simulink model "RefModel_Task"  (R2015b)
settings: configuration reference "CenterOutReachConfigSet" (kept outside this file)
undefined symbols (not defined in the file or in its folder): SimulinkParameter_TunableConditionRepeats, SimulinkParameter_TunableConditions, SimulinkParameter_TunableDataLoggerInfo, SimulinkParameter_TunableNextTrialId, SimulinkParameter_TunableParam, SimulinkParameter_TunableTaskControl
libraries: libBusSerialize x7, libUtilities x1, dspsrcs4 x1
(part 2 of 3)

== stateflow chart RefModel_Task/Task Stateflow ==
  state TaskTimeoutContainer [parallel]
    settings: executionOrder=1
    state TaskNotRunning
      en:
      TD.taskRunning = uint8(0);
      JuiceRelease = uint8(0);
      if TaskControl.controlImaging
      % if we were imaging, pause it
      scopeCommand = ScopeCommand.StopImaging;
      send(SendScope);
      end
      ex:
      TD.taskRunning = uint8(1);
      state TaskPaused
        en:
        state = TaskState.TaskPaused;
        displayCommand = DisplayCommand.TaskPaused;
        send(SendDisplay);
      state TaskPurgatory
        en:
        TD.inPurgatory = uint8(1);
        TD.purgatoryTimeRemaining = P.purgatoryTime;
        state = TaskState.TaskPurgatory;
        TD.consecutiveNoStarts = uint16(0);
        displayCommand = DisplayCommand.TaskTimeout;
        send(SendDisplay);
        du:
        TD.purgatoryTimeRemaining = TD.purgatoryTimeRemaining - uint32(1);
        ex:
        TD.inPurgatory = uint8(0);
    state Task
      state TaskFlow [parallel]
        du:
        computeHandState();
        ex:
        send(AbortJuice, JuiceToggle);
        settings: executionOrder=1
        state InitTrial
          en:
          send(TrialStart);
          send(PhotoboxReset, PhotoboxEvents);
          TD.taskRunning = uint8(1);
          % this counter will be reset to zero when the appropriate
          % point in the trial has been reached
          TD.consecutiveNoStarts = TD.consecutiveNoStarts + uint16(1);
          displayCommand = DisplayCommand.InitTrial;
          send(SendDisplay);
          if C.hasImaging && TaskControl.controlImaging
          TD.imagingThisTrial = uint8(1);
          scopeCommand = ScopeCommand.NextTrial;
          send(SendScope);
          scopeCommand = ScopeCommand.StartImagingOnTrigger;
          send(SendScope);
          else
          TD.imagingThisTrial = uint8(0);
          end
          state = TaskState.InitTrial;
          resetTrialData();
        state StartTask
          en:
          state = TaskState.StartTask;
          displayCommand = DisplayCommand.StartTask;
          send(SendDisplay);
        state CenterAcquireHold
          state CenterAcquireLogic [parallel]
            settings: executionOrder=1
            state WaitCenterAcquire
              en:
              state = TaskState.WaitCenterAcquire;
              displayCommand = DisplayCommand.CenterOnset;
              send(SendDisplay);
              eventCode = TaskEvent.CenterOnset;
              send(SendEvent);
            state WaitCenterSettle
              en:
              state = TaskState.WaitCenterSettle;
              displayCommand = DisplayCommand.CenterAcquired;
              send(SendDisplay);
              eventCode = TaskEvent.CenterAcquired;
              send(SendEvent);
              ex:
              % Establish hold window for td.isHolding
              TD.holdXCenter = HandBus.handX;
              TD.holdYCenter = HandBus.handY;
            state CenterUnacquire
              en: displayCommand = DisplayCommand.CenterUnacquired;
              send(SendDisplay);
              eventCode = TaskEvent.CenterUnacquired;
              send(SendEvent);
            state WaitCenterHold
              en:
              state = TaskState.WaitCenterHold;
              displayCommand = DisplayCommand.CenterSettled;
              send(SendDisplay);
              eventCode = TaskEvent.CenterSettled;
              send(SendEvent);
              % trigger imaging just before TargetOnset
              on after(P.timeCenterHold - P.timeImagingStartBeforeTargetOnset, tick):
              if TD.imagingThisTrial
              scopeCommand = ScopeCommand.StartTrialImaging;
              send(SendScope);
              end
            state CenterHeld
              en:
              displayCommand = DisplayCommand.CenterHeld;
              send(SendDisplay);
              eventCode = TaskEvent.CenterHeld;
              send(SendEvent);
              if P.timeJuiceCenter > 0
              TD.juiceNumDrops = uint16(1);
              TD.juiceDropSize = uint16(P.timeJuiceCenter);
              send(SendJuice, JuiceToggle);
              end
            WaitCenterAcquire -> WaitCenterSettle [order 1] : [TD.isTouchingCenter == 1]
            CenterUnacquire -> WaitCenterAcquire
            WaitCenterSettle -> WaitCenterHold : after(P.timeCenterSettle,tick)
                | % Wait for settling before enforcing hold
            (junction 2183) -> CenterUnacquire [order 2]
            (junction 2186) -> CenterUnacquire [order 2]
            WaitCenterHold -> (junction 2183) [order 1] : [~HandBus.handSeen]
                | % Missing hand position
            WaitCenterHold -> (junction 2186) [order 3] : [~TD.isHoldingCenter]
                | % Moved during center hold = hold - 1> fail trial
            WaitCenterHold -> CenterHeld [order 2] : after(P.timeCenterHold,tick)
                | % Held center
        state ForceNewCondition
          en:
          TD.getNewTrialParams = uint8(1);
        state TrialFailure
          en:
          TD.success = uint8(0);
          if TD.imagingThisTrial
          scopeCommand = ScopeCommand.EndTrialImaging;
          send(SendScope);
          end
          state FailureCenterAcquire % never got to center
            en:
            TD.substantiveFailure = uint8(0);
            TD.getNewTrialParams = uint8(0);
            state = TaskState.FailureCenterAcquire;
            displayCommand = DisplayCommand.FailureCenterFlyAway;
            send(SendDisplay);
            eventCode = TaskEvent.FailureToAcquireCenter;
            send(SendEvent);
          state FailureComputeITI
            en:
            if P.repeatUntilSuccess
            TD.getNewTrialParams = uint8(0);
            end
            TD.failureCode = state;
            computeFailureITI();
            % print failure message to screen
            coder.ceval('printf', ['Failure: %s' 10 0], ...
            [enumToString_TaskState(state) uint8(0)]);
          state FailureHandNotSeen % lost hand position during trial
            en:
            TD.substantiveFailure = uint8(0);
            TD.getNewTrialParams = uint8(1);
            state = TaskState.FailureHandNotSeen;
            displayCommand = DisplayCommand.FailureCenterFlyAway;
            send(SendDisplay);
            eventCode = TaskEvent.FailureHandNotSeen;
            send(SendEvent);
            % print warning message to screen
            coder.ceval('printf', ['WARNING: HAND NOT SEEN' 10 0]);
          state FailureCenterHold % moved while holding
            en:
            TD.substantiveFailure = uint8(0);
            TD.getNewTrialParams = uint8(0);
            state = TaskState.FailureCenterHold;
            displayCommand = DisplayCommand.FailureCenterFlyAway;
            send(SendDisplay);
            eventCode = TaskEvent.FailureBrokeCenterHold;
            send(SendEvent);
          state FailureDelayMove % moved during delay
            en:
            TD.substantiveFailure = uint8(0);
            TD.getNewTrialParams = uint8(1);
            state = TaskState.FailureDelayMove;
            displayCommand = DisplayCommand.FailureTargetFlyAway;
            send(SendDisplay);
            eventCode = TaskEvent.FailureBrokeCenterHoldDelay;
            send(SendEvent);
          state FailureRTTooFast % moved too early post go-cue
            en:
            TD.substantiveFailure = uint8(0);
            TD.getNewTrialParams = uint8(1);
            state = TaskState.FailureRTTooFast;
            displayCommand = DisplayCommand.FailureTargetFlyAway;
            send(SendDisplay);
            eventCode = TaskEvent.FailureRTTooFast;
            send(SendEvent);
          state FailureRTTooSlow % didn't move early enough post go-cue
            en:
            TD.substantiveFailure = uint8(0);
            TD.getNewTrialParams = uint8(1);
            state = TaskState.FailureRTTooSlow;
            displayCommand = DisplayCommand.FailureTargetFlyAway;
            send(SendDisplay);
            eventCode = TaskEvent.FailureRTTooSlow;
            send(SendEvent);
          state FailureTargetAcquire % didn't get target in time
            en:
            TD.substantiveFailure = uint8(1);
            TD.getNewTrialParams = uint8(1);
            state = TaskState.FailureTargetAcquire;
            displayCommand = DisplayCommand.FailureTargetFlyAway;
            send(SendDisplay);
            eventCode = TaskEvent.FailureToAcquireTarget;
            send(SendEvent);
          state FailureTargetHold % moved while holding target
            en:
            TD.substantiveFailure = uint8(1);
            TD.getNewTrialParams = uint8(1);
            state = TaskState.FailureTargetHold;
            displayCommand = DisplayCommand.FailureTargetFlyAway;
            send(SendDisplay);
            eventCode = TaskEvent.FailureToAcquireTarget;
            send(SendEvent);
          state FailurePeakVelocityTooLow % reach too slow
            en:
            TD.substantiveFailure = uint8(1);
            TD.getNewTrialParams = uint8(1);
            state = TaskState.FailureLowPeakVelocity;
            displayCommand = DisplayCommand.FailureTargetFlyAway;
            send(SendDisplay);
            eventCode = TaskEvent.FailureLowPeakVelocity;
            send(SendEvent);
          FailureCenterAcquire % never got to center -> (junction 1353)
          (junction 1353) -> FailureComputeITI : after(1,tick)
          FailureHandNotSeen % lost hand position during trial -> (junction 1353)
          FailurePeakVelocityTooLow % reach too slow -> (junction 1353)
          FailureCenterHold % moved while holding -> (junction 1353)
          FailureDelayMove % moved during delay -> (junction 1353)
          FailureTargetHold % moved while holding target -> (junction 1353)
          FailureRTTooFast % moved too early post go-cue -> (junction 1353)
          FailureRTTooSlow % didn't move early enough post go-cue -> (junction 1353)
          FailureTargetAcquire % didn't get target in time -> (junction 1353)
        state DelayPeriodGoCue
          state GoCue
            state GoCueZeroDelay
              en:
              state = TaskState.GoCueZeroDelay;
              TD.timeTargetOnsetCommand = GlobalClock;
              TD.timeGoCueCommand = GlobalClock;
              displayCommand = DisplayCommand.GoCueZeroDelay;
              send(SendDisplay);
              eventCode = TaskEvent.TargetOnsetCommand;
              send(SendEvent);
              eventCode = TaskEvent.GoCueCommand;
              send(SendEvent);
            state GoCueNonZeroDelay
              en:
              state = TaskState.GoCueNonZeroDelay;
              TD.timeGoCueCommand = GlobalClock;
              displayCommand = DisplayCommand.GoCueNonZeroDelay;
              send(SendDisplay);
              eventCode = TaskEvent.GoCueCommand;
              send(SendEvent);
          state SetTargetInfo
            en:
            TD.targetXCurrent = C.targetX;
            TD.targetYCurrent = C.targetY;
            TD.targetSizeCurrent = C.targetSize;
          state DelayPeriod
            en:
            state = TaskState.DelayPeriod;
            TD.timeTargetOnsetCommand = GlobalClock;
            displayCommand = DisplayCommand.DelayPeriodStart;
            send(SendDisplay);
            eventCode = TaskEvent.TargetOnsetCommand;
            send(SendEvent);
          state WaitMoveOnset
            en:
            state = TaskState.WaitMoveOnset;
            if P.imageDecoderDebugDisplayMode
            end
            du:
            TD.rt = GlobalClock - TD.timeGoCue; % detected by photobox
            TD.rtNominal = GlobalClock - TD.timeGoCueCommand; % not detected by photobox
            ex:
            TD.timeMove = GlobalClock;
            TD.rt = GlobalClock - TD.timeGoCue; % not detected by photobox
            TD.rtNominal = GlobalClock - TD.timeGoCueCommand; % not detected by photobox
            displayCommand = DisplayCommand.MoveOnset;
            send(SendDisplay)
            eventCode = TaskEvent.MoveOnsetOnline;
            send(SendEvent);
          (default) -> SetTargetInfo
          SetTargetInfo -> GoCueZeroDelay [order 1] : [~C.hasCenterTouch || C.delayNominal == 0]
              | % Target Only Zero Delay
          SetTargetInfo -> DelayPeriod [order 2] : % Non-zero Delay
          DelayPeriod -> GoCueNonZeroDelay [order 2] : after(C.delayNominal, tick)
              | % Delay period over
          GoCue -> WaitMoveOnset : after(1,tick)
          WaitMoveOnset -> (junction 1269) [order 2] : [~TD.isHoldingCenter]
              | % Move from center
        state RequestNewTrial
          en: send(GetNewTrial);
        state TargetAcquireHold
          state WaitTargetAcquire
            en:
            state = TaskState.WaitTargetAcquire;
          state WaitTargetSettle
            en:
            % count as initiated the trial (for ~hasCenterTouch)
            TD.consecutiveNoStarts = uint16(0);
            state = TaskState.WaitTargetSettle;
            displayCommand = DisplayCommand.TargetAcquired;
            send(SendDisplay);
            eventCode = TaskEvent.TargetAcquired;
            send(SendEvent);
          state TargetUnacquire
            en: displayCommand = DisplayCommand.TargetUnacquired;
            send(SendDisplay);
            eventCode = TaskEvent.TargetUnacquired;
            send(SendEvent);
          state WaitTargetHold
            en:
            % Establish the hold window around current hand pos
            TD.holdXTarget = HandBus.handX;
            TD.holdYTarget = HandBus.handY;
            state = TaskState.WaitTargetHold;
            % Send TargetSettled
            displayCommand = DisplayCommand.TargetSettled;
            send(SendDisplay);
            eventCode = TaskEvent.TargetSettled;
            send(SendEvent);
            % optionally juice during target hold
            if C.juiceDuringTargetHold
            TD.juiceNumDrops = uint16(50);
            TD.juiceDropSize = uint16(P.targetHoldJuiceSize);
            TD.juiceDropInterval = uint16(P.targetHoldJuiceInterval);
            send(SendJuice, JuiceToggle);
            end
            ex:
            displayCommand = DisplayCommand.TargetHeld;
            send(SendDisplay);
            eventCode = TaskEvent.TargetHeld;
            send(SendEvent);
            send(AbortJuice, JuiceToggle);
          WaitTargetAcquire -> WaitTargetSettle [order 2] : [TD.isTouchingTarget]
              | % Target Acquired
          TargetUnacquire -> WaitTargetAcquire
          (junction 2191) -> TargetUnacquire [order 2] : % allow target reacquire
          WaitTargetSettle -> WaitTargetHold : after(P.timeTargetSettle, tick)
          WaitTargetHold -> (junction 2191) [order 2] : [~TD.isHoldingTarget]
              | % Moved during TargetHold
        state ITI
          en:
          send(TrialEnd);
          state = TaskState.ITI;
          displayCommand = DisplayCommand.ITI;
          send(SendDisplay);
          send(TrialITI);
        state Success
          en:
          state = TaskState.Success;
          TD.success = uint8(1);
          TD.getNewTrialParams = uint8(1);
          if TD.imagingThisTrial
          scopeCommand = ScopeCommand.EndTrialImaging;
          send(SendScope);
          end
          computeRewardAndITI();
          send(SendJuice, JuiceToggle);
          displayCommand = DisplayCommand .Success;
          send(SendDisplay);
          eventCode = TaskEvent.Success;
          send(SendEvent);
          coder.ceval('printf', ['Success: giving %u ms juice' 10 0], ...
          TD.juiceTimeTotal);
        (default) -> StartTask
        RequestNewTrial -> InitTrial : after(1, tick)
        InitTrial -> (junction 2180) : after(1,tick)
        (junction 2180) -> DelayPeriodGoCue [order 2] : [~C.hasCenterTouch]
        StartTask -> ForceNewCondition : after(1,tick)
        ForceNewCondition -> RequestNewTrial
        (junction 1387) -> RequestNewTrial [order 2]
        ITI -> (junction 1387) : after(TD.iti,tick)
            | % Wait ITI
        Success -> ITI : after(P.timeRewardFeedback,tick)
            | % Wait for target white flash
        WaitTargetAcquire -> FailurePeakVelocityTooLow % reach too slow [order 3] : % Peak Velocity Too Low
            | [TD.peakVelocityTowardsTargetTooLow && ...
            | C.enforceMinPeakVelocity]
        (junction 2183) -> FailureHandNotSeen % lost hand position during trial [order 1] : [~P.allowReacquireCenter]
            | % Fail trial hand not seen
        (junction 1269) -> WaitTargetAcquire [order 1] : [TD.rtNominal >= P.rtMin]
            | % RT acceptable
        FailureComputeITI -> ITI : after(TD.timeFailureFeedback,tick)
        WaitCenterAcquire -> FailureCenterAcquire % never got to center [order 2] : after(P.timeCenterAcquire,tick)
            | % Did not acquire center
        (junction 2186) -> FailureCenterHold % moved while holding [order 1] : [~P.allowReacquireCenter]
            | % Fail trial didn't hold center
        WaitTargetAcquire -> FailureTargetAcquire % didn't get target in time [order 1] : after(P.timeTargetAcquire, tick)
            | % Did not acquire target
        (junction 2180) -> WaitCenterAcquire [order 1] : [C.hasCenterTouch]
        (junction 2191) -> FailureTargetHold % moved while holding target [order 1] : [~P.allowReacquireTarget]
            | % Fail trial left target hold
        DelayPeriod -> FailureDelayMove % moved during delay [order 1] : [~TD.isHoldingCenter]
            | % Moved during delay
        CenterHeld -> DelayPeriodGoCue
        WaitTargetHold -> Success [order 1] : after(P.timeTargetHold, tick)
            | % Held target
        DelayPeriodGoCue -> FailureHandNotSeen % lost hand position during trial : [~HandBus.handSeen && C.hasCenterTouch && ~P.allowHandNotSeen]
            | % Missing hand position
        (junction 1269) -> FailureRTTooFast % moved too early post go-cue [order 2] : [TD.rtNominal < P.rtMin && C.hasCenterTouch]
            | % RT too fast
        TargetAcquireHold -> FailureHandNotSeen % lost hand position during trial : [~HandBus.handSeen && C.hasCenterTouch && ~P.allowHandNotSeen]
            | % Missing hand position
        WaitMoveOnset -> FailureRTTooSlow % didn't move early enough post go-cue [order 1] : after(P.rtMax,tick)  [C.hasCenterTouch]
            | % RT too slow
      state JuiceToggle [parallel]
        settings: executionOrder=3
        state JuiceDeliverDrops
          en:
          TD.juiceDropsRemaining = TD.juiceNumDrops;
          ex:
          JuiceRelease = uint8(0);
          state JuiceDropInterval
            en:
            JuiceRelease = uint8(0);
            TD.juiceDropsRemaining = TD.juiceDropsRemaining - uint16(1);
          state JuiceDropReleasing
            en:
            JuiceRelease  = uint8(1);
          (default) -> JuiceDropReleasing
          JuiceDropReleasing -> JuiceDropInterval : after(TD.juiceDropSize, tick)
          JuiceDropInterval -> JuiceDropReleasing [order 2] : after(TD.juiceDropInterval - TD.juiceDropSize, tick)
        state Off
          en:
          JuiceRelease = uint8(0);
        Off -> JuiceDropReleasing : SendJuice
        JuiceDropInterval -> Off [order 1] : [TD.juiceDropsRemaining < 1 || TD.juiceDropsRemaining > 10]
        JuiceDeliverDrops -> Off : AbortJuice
        (default) -> Off
      state PhotoboxEvents [parallel]
        settings: executionOrder=2
        state PhotoboxLogic
          state PhotoboxOnZeroDelayTrial
            en:
            eventCode = TaskEvent.TargetOnset;
            TD.timeTargetOnset = GlobalClock;
            send(SendEvent);
          state PhotoboxSendGoCue
            en:
            eventCode = TaskEvent.GoCue;
            TD.timeGoCue = GlobalClock;
            TD.delay = TD.timeGoCue - TD.timeTargetOnset;
            send(SendEvent);
            send(ImagingGoCue, ImagingEvents);
          state PhotoboxOnDelayTrial
            en:
            eventCode = TaskEvent.TargetOnset;
            TD.timeTargetOnset = GlobalClock;
            send(SendEvent);
          state PhotoboxWaitOn
          PhotoboxLogic -> PhotoboxWaitOn : PhotoboxReset
          PhotoboxOnZeroDelayTrial -> PhotoboxSendGoCue
          PhotoboxOnDelayTrial -> PhotoboxSendGoCue : [Photobox==0]
          (junction 1713) -> PhotoboxOnZeroDelayTrial [order 2] : [C.delayNominal == 0]
          PhotoboxSendGoCue -> PhotoboxWaitOn : [Photobox==0]
          (default) -> PhotoboxWaitOn
          (junction 1713) -> PhotoboxOnDelayTrial [order 1] : [C.delayNominal > 0]
          PhotoboxWaitOn -> (junction 1713) : [Photobox==1]
      state ImagingEvents [parallel]
        settings: executionOrder=4
        state waitTSkip
          entry: TD.useNextFrame = uint8(0);
        state PresentDecodeTestObject
          en:
          displayCommand = DisplayCommand.ImageDecodeTestObject;
          send(SendDisplay);
        state Wait
          en:
          TD.useNextFrame = uint8(0);
        state waitTInt
          en:
          TD.useNextFrame = uint8(1);
        state DecodeComplete
          en:
          TD.decodeComplete = uint8(1);
          if P.conditionsToDecode(C.conditionId)
          eventCode = TaskEvent.DecodeComplete;
          send(SendEvent);
          if (D.decodeConditionId == C.conditionId)
          TD.decodeSuccess = uint8(1);
          displayCommand = DisplayCommand.DecodeSuccess;
          send(SendDisplay);
          coder.ceval('printf', ['--decode success, cond: %u, decode cond: %u:' 10 0], ...
          C.conditionId, D.decodeConditionId);
          else
          TD.decodeSuccess = uint8(0);
          displayCommand = DisplayCommand.DecodeFail;
          send(SendDisplay);
          coder.ceval('printf', ['--decode fail, cond: %u, decode cond: %u:' 10 0], ...
          C.conditionId, D.decodeConditionId);
          end
          else
          coder.ceval('printf', ['--decode ignore' 10 0]);
          end
        state stopFrameAcquire
          entry: TD.useNextFrame = uint8(0);
          displayCommand = DisplayCommand.ImageDecodeTestObjectHide;
          send(SendDisplay);
        TaskTimeoutContainer.Task.ImagingEvents.Wait -> waitTSkip : ImagingGoCue
        waitTSkip -> PresentDecodeTestObject : after(P.frameSkipTime-80,tick)
        (default) -> TaskTimeoutContainer.Task.ImagingEvents.Wait
        stopFrameAcquire -> TaskTimeoutContainer.Task.ImagingEvents.Wait [order 2] : [P.imageDecoderTraining == 1]
        TaskTimeoutContainer.Task.ImagingEvents.DecodeComplete -> TaskTimeoutContainer.Task.ImagingEvents.Wait
        PresentDecodeTestObject -> waitTInt : after(80, tick)
        waitTInt -> stopFrameAcquire : after(P.frameIntegrationTime,tick)
        stopFrameAcquire -> TaskTimeoutContainer.Task.ImagingEvents.DecodeComplete [order 1] : % last update after
            | % acquisition complete
            | [D.decodeConditionId ~= 0]
      state DecodeEvents [parallel] [commented out]
        state DecodeComplete [commented out]
          en:
          TD.decodeComplete = uint8(1);
          if (decodeConditionId == C.conditionId)
          TD.decodeSuccess = uint8(1);
          displayCommand = DisplayCommand.DecodeSuccess;
          send(SendDisplay);
          else
          TD.decodeSuccess = uint8(0);
          displayCommand = DisplayCommand.DecodeFail;
          send(SendDisplay);
          end
        state Wait [commented out]
        (default) -> TaskTimeoutContainer.Task.DecodeEvents.Wait [commented out]
        TaskTimeoutContainer.Task.DecodeEvents.Wait -> TaskTimeoutContainer.Task.DecodeEvents.DecodeComplete [commented out] : [decodeConditionId ~= 0]
        TaskTimeoutContainer.Task.DecodeEvents.DecodeComplete -> TaskTimeoutContainer.Task.DecodeEvents.Wait [commented out] : [decodeConditionId == 0]
    (default) -> TaskPaused
    Task -> TaskPaused : [TaskControl.runTask == 0]
        | % Task paused
    TaskPaused -> StartTask : [TaskControl.runTask == 1]
        | % Task started
    (junction 1387) -> TaskPurgatory [order 1] : [TaskControl.autoTimeoutActive && ...
        | TD.consecutiveNoStarts >= P.purgatoryConsecutiveNoStarts]
        | % Enter purgatory if too many no-starts
    TaskPurgatory -> ForceNewCondition : [TaskControl.endTimeoutNow || ...
        |  TaskControl.autoTimeoutActive==0 || ...
        |  TD.purgatoryTimeRemaining == 0]
        | % Return from Purgatory
  data: tf function_output uint8 size=1; cX function_input double; cY function_input double; diameter function_input double; distance function_output double size=1; velocity function_output double size=1; acceleration function_output double size=1; lateralDistance function_output; lateralVelocity function_output; lateralAcceleration function_output; JuiceRelease output uint8 size=1; TaskControl input Bus: TaskControlBus size=1; P input Bus: ParamBus size=1; state local Enum: TaskState size=1; C input Bus: ConditionFixedBus size=1; GlobalClock input uint32 size=1; displayCommand output Enum: DisplayCommand size=1; HandBus input Bus: HandBus size=1; Photobox input size=1; TD data_store_memory; eventCode output Enum: TaskEvent size=1; scopeCommand output Enum: ScopeCommand size=1; D input Bus: DecoderBus size=1
  events: AbortJuice local FUNCTION_CALL_EVENT; SendJuice local FUNCTION_CALL_EVENT; ImagingGoCue local FUNCTION_CALL_EVENT; SendDisplay output FUNCTION_CALL_EVENT; SendEvent output FUNCTION_CALL_EVENT; SendScope output FUNCTION_CALL_EVENT; TrialStart output FUNCTION_CALL_EVENT; TrialEnd output FUNCTION_CALL_EVENT; TrialITI output FUNCTION_CALL_EVENT; GetNewTrial output FUNCTION_CALL_EVENT; PhotoboxReset local FUNCTION_CALL_EVENT
  function tf = isTouchingCircle(cX, cY, diameter):
    | function tf = isTouchingCircle(cX, cY, diameter)
    | 
    | x = HandBus.handX;
    | y = HandBus.handY;
    | z = HandBus.handZ;
    | 
    | if HandBus.handSeen && HandBus.handTouching && ...
    |   (x - cX)^2 + (y - cY)^2 < (diameter/2)^2
    |     tf = uint8(1);
    | else
    |     tf = uint8(0);
    | end
  function resetTrialData:
    | function resetTrialData()
    |     TD.peakVelocityTowardsTarget = 0;
    |     TD.timeInitTrial = GlobalClock;
    |     TD.timeGoCueCommand = uint32(0);
    |     TD.timeGoCue = uint32(0);
    |     TD.timeTargetOnsetCommand = uint32(0);
    |     TD.timeTargetOnset = uint32(0);
    |     TD.timeMove = uint32(0);
    |     TD.rt = uint32(0);
    |     TD.rtNominal = uint32(0);
    |     TD.delay = uint32(0);
    |     TD.iti = uint32(0);
    |     TD.holdXCenter = NaN;
    |     TD.holdYCenter = NaN;
    |     TD.holdXTarget = NaN;
    |     TD.holdYTarget = NaN;
    |     TD.targetXCurrent = 0;
    |     TD.targetYCurrent = 0;
    |     TD.targetSizeCurrent = 0;
    |     TD.isTouchingTarget = uint8(0);
    |     TD.substantiveFailure = uint8(0);
    |     TD.moveOnsetThreshOccurred = uint8(0);
    |     TD.peakVelocityTowardsTarget = 0;
    |     TD.peakAccelerationTowardsTarget = 0;    
    |     TD.postPeakMinAccelerationTowardsTarget = 0;
    |     TD.useNextFrame = uint8(0);
    |     TD.decodeComplete = uint8(0);
    |     TD.decodeSuccess = uint8(0);
    |     TD.isDecodeCondition = uint8(P.conditionsToDecode(C.conditionId));
    |     
    | end
  function computeHandState:
    | function computeHandState()
    | 
    | if state ~= TaskState.InitTrial
    |     % determine if we're within the center hold windows
    |     TD.isTouchingCenter = isTouchingCircle(C.centerX, C.centerY, P.centerSize + P.acceptanceWindowPadding);
    |     TD.isHoldingCenter = uint8(isTouchingCircle(TD.holdXCenter, TD.holdYCenter, P.centerHoldWindowSize) && ~HandBus.handMoving);
    |  
    |     % determine if we're touching the target
    |     TD.isTouchingTarget = isTouchingCircle(TD.targetXCurrent, TD.targetYCurrent, TD.targetSizeCurrent + P.acceptanceWindowPadding);
    |     TD.isHoldingTarget = uint8(isTouchingCircle(TD.holdXTarget, TD.holdYTarget, P.targetHoldWindowSize) && ~HandBus.handMoving);
    | 
    |     if TD.timeGoCueCommand > 0
    |         % figure out our distance/velocity in direction of target
    |         [TD.distanceTowardsTarget, TD.velocityTowardsTarget, TD.accelerationTowardsTarget, ...
    |          TD.lateralDistance, TD.lateralVelocity, TD.lateralAcceleration] = ...
    |             computeProgressTowardsTarget();
    |         
    |         if ~TD.moveOnsetThreshOccurred && ...
    |                 TD.velocityTowardsTarget >= P.velocityTowardsTargetThresh && ...
    |                 TD.distanceTowardsTarget >= P.distanceTowardsTargetThresh
    |             TD.moveOnsetThreshOccurred = uint8(1);
    |             eventCode = TaskEvent.MoveOnsetThresh;
    |             send(SendEvent);
    |         end
    |         
    |         % during movement, track velocity and acceleration, also log double
    |         % accelerations, i.e. stops and starts
    |         if TD.moveOnsetThreshOccurred && ~TD.isTouchingTarget
    |             % update peak velocity after move onset
    |             if TD.peakVelocityTowardsTarget < TD.velocityTowardsTarget
    |                 TD.peakVelocityTowardsTarget = TD.velocityTowardsTarget;
    |             end
    | 
    |             % update peak acceleration after move onset
    |             if TD.moveOnsetThreshOccurred && TD.peakAccelerationTowardsTarget < TD.accelerationTowardsTarget
    |                 TD.peakAccelerationTowardsTarget = TD.accelerationTowardsTarget;
    |             end
    |         
    |             % wait for sufficient initial acceleration, then detect decleration
    |             if TD.peakAccelerationTowardsTarget > P.threshAcceleration && ...
    |                 TD.accelerationTowardsTarget < P.decelerationThreshRatio * TD.peakAccelerationTowardsTarget
    |                 % we've decelerated below threshold*peak
    |                 if ~TD.deceleratedBelowThresh
    |                     % store a good initial value since it starts out at 0 otherwise
    |                     TD.postPeakMinAccelerationTowardsTarget = TD.accelerationTowardsTarget;
    |                 end
    |                 TD.deceleratedBelowThresh = uint8(1);
    |             end
    |             
    |              % if our velocity has dropped now that we've decelerated, check whether peak velocity
    |              % was high enough
    |              if TD.peakAccelerationTowardsTarget > P.threshAcceleration && ...
    |                  TD.velocityTowardsTarget < P.decelerationThreshRatio * TD.peakVelocityTowardsTarget && ...
    |                  TD.peakVelocityTowardsTarget < P.minPeakVelocityTowardsTarget
    |                  TD.peakVelocityTowardsTargetTooLow = uint8(1);
    |              end
    |             
    |             % track the minimum acceleration after decelerating
    |             if TD.deceleratedBelowThresh && TD.accelerationTowardsTarget < TD.postPeakMinAccelerationTowardsTarget
    |                 TD.postPeakMinAccelerationTowardsTarget = TD.accelerationTowardsTarget;
    |             end
    |         end
    |     else
    |         TD.peakVelocityTowardsTarget = 0;
    |         TD.peakAccelerationTowardsTarget = 0;
    |         TD.postPeakMinAccelerationTowardsTarget = 0;
    |         TD.deceleratedBelowThresh = uint8(0);
    |         TD.peakVelocityTowardsTargetTooLow = uint8(0);
    |     end    
    |     
    | end
  function [distance, velocity, acceleration, lateralDistance, lateralVelocity, lateralAcceleration] = computeProgressTowardsTarget:
    | function [distance, velocity, acceleration, lateralDistance, lateralVelocity, lateralAcceleration] = computeProgressTowardsTarget()
    | % given the Condition and hand position, compute whether
    | % the hand is in the target. Score is a double that ranges from 0 to 1, 
    | % which will indicate some metric of lateral deviation
    | 
    | hx = HandBus.handX;
    | hy = HandBus.handY;
    | vx = HandBus.handVelocityX;
    | vy = HandBus.handVelocityY;
    | ax = HandBus.handAccelerationX;
    | ay = HandBus.handAccelerationY;
    | cx = C.centerX;
    | cy = C.centerY;
    | size = TD.targetSizeCurrent;
    | 
    | % translate/rotate target and hand coordinates so that target is straight upwards, i.e. at
    | % X: -width/2 to +width/2
    | % Y: targetDistance +/- targetDepth/2
    | thetaOrientation = C.targetDirection - pi/2;
    | rot = [ cos(thetaOrientation), sin(thetaOrientation); ...
    |        -sin(thetaOrientation), cos(thetaOrientation)];
    | rotHand = rot * [hx - cx; hy - cy];
    | rhx = rotHand(1);
    | rhy = rotHand(2);
    | rotVel =  rot * [vx; vy];
    | rvx = rotVel(1);
    | rvy = rotVel(2);
    | 
    | rotAcc = rot * [ax; ay];
    | rax = rotAcc(1);
    | ray = rotAcc(2);
    | 
    | distance = 0;
    | velocity = 0;
    | acceleration = 0;
    | lateralDistance = 0;
    | lateralVelocity = 0;
    | lateralAcceleration = 0;
    | 
    | if HandBus.handSeen && HandBus.handTouching
    |     distance = rhy;
    |     velocity = rvy;
    |     acceleration = ray;
    |     lateralDistance = rhx;
    |     lateralVelocity = rvx;
    |     lateralAcceleration = rax;
    | end
  function computeRewardAndITI:
    | function computeRewardAndITI()
    | % split juice into discrete drops and compute the pulse train to play as
    | % the reward signal
    | 
    | if TD.decodeSuccess
    |     TD.juiceTimeTotal = uint32(P.timeJuiceDecodeSuccess);
    | else
    |     TD.juiceTimeTotal = uint32(P.timeJuice); 
    | end
    | TD.juiceNumDrops = uint16(1);
    | TD.juiceDropSize = uint16(TD.juiceTimeTotal);
    | 
    | TD.juiceDropInterval = uint16(400);
    | 
    | TD.iti = P.itiSuccess;
    | 
    | end
  function computeFailureITI:
    | function computeFailureITI()
    | 
    | TD.timeFailureFeedback = P.timeFailureFeedback;
    | TD.iti = P.itiFailure;
    | TD.juiceTimeTotal = uint32(0);
    | 
    | end

== matlab function RefModel_Task/Tunable Data Logger Info/Deserialize Bus Parameter ==
  data: valAsDouble input double; bus output Bus: DataLoggerInfoBus size=1; update output uint8 size=1; allowPending input uint8 size=1; receivedInvalid output uint8 size=1
function [bus, update, receivedInvalid] = deserializeBusParameter(valAsDouble, allowPending)
%#codegen

    % typecast to bytes
    valAsBytes = typecast(valAsDouble, 'uint8');

    % use the first byte as updateCounter, check for whether counter has been incremented
    thisCounter = valAsBytes(1);
    persistent pLastCounter;
    if isempty(pLastCounter)
        pLastCounter = thisCounter;
    end
    if pLastCounter ~= thisCounter
        recvUpdate = uint8(1);
        pLastCounter = thisCounter;
    else
        recvUpdate = uint8(0);
    end
    startOffset = 2;

    % external cached output for when allowPending 
    persistent pBusOut;
    if isempty(pBusOut)
        pBusOut = initializeBus_DataLoggerInfoBus();
    end

    % parse incoming bytes if allowing updates
    receivedInvalid = uint8(0);
    if allowPending
        [bus, valid] = deserializeBus_DataLoggerInfoBus(valAsBytes, startOffset);
        if valid
            % update internal cache
            pBusOut = bus;
        else
            % don't update internal cache, output internal cache
            bus = pBusOut;
            receivedInvalid = uint8(1);
            recvUpdate = uint8(0);
        end
    else
        bus = pBusOut;
    end

    % track whether we have a pending update
    persistent pPending;
    if isempty(pPending), pPending = uint8(0); end
    if recvUpdate
        if allowPending
            % update goes out immediately
            update = uint8(1);
            pPending = uint8(0);
        else
            % queue pending update
            update = uint8(0);
            pPending = uint8(1);
        end
    else
        if allowPending
            % release pending
            update = pPending;
            pPending = uint8(0);
        else
            % do nothing
            update = uint8(0);
        end
    end

    % reset fields marked with .resetImmediately immediately after update
    if ~update

    end
end

== matlab function RefModel_Task/Tunable Condition Repeats/Deserialize Parameter ==
  data: valAsDouble input double; value output uint16 size=[20 1]; update output uint8 size=1
function [value, update] = deserializeParameter(valAsDouble)
%#codegen

valAsBytes = typecast(valAsDouble, 'uint8');

% check for whether counter has been incremented
thisCounter = valAsBytes(1);
persistent pLastCounter;
if isempty(pLastCounter)
    pLastCounter = thisCounter;
end
if pLastCounter ~= thisCounter
    update = uint8(1);
    pLastCounter = thisCounter;
else
    update = uint8(0);
end

% typecast and reshape the value
value = reshape(typecast(valAsBytes(double(2):double(41)), 'uint16'), [20 1]);

== matlab function RefModel_Task/Add dynamic properties to condition ==
  data: newTrial input; C input Bus: ConditionBus size=1; Cout output Bus: ConditionBus size=1; randUnifInput input double size=1; taskControl input
function Cout = modifyCondition(newTrial, C, randUnifInput, taskControl)
%#codegen

% update the random input when newTrial
persistent pRandInput
if isempty(pRandInput) || newTrial
    pRandInput = randUnifInput;
end
    
% add random delay period
Cout = modifyDynamicConditionAttributes(C, pRandInput);

% determine whether to image this trial
persistent pCounter;
if isempty(pCounter)
    pCounter = uint32(0);
end
persistent pImage;
if isempty(pImage)
    pImage = uint8(0);
end

if newTrial
    pCounter = pCounter + 1;
    % image every nth trial if we're controlling imaging and savingData
    if taskControl.controlImaging && ...
            pCounter >= taskControl.imageEveryNthTrial
        pCounter = uint32(0);
        pImage = uint8(1);
    else
        pImage = uint8(0);
    end
end
Cout.hasImaging = pImage;

if newTrial && numel(C.conditionDesc) > 0
    if ~Cout.hasImaging
        coder.ceval('printf', ['C%d: %s delay %.0f ms' 10 0], ...
            Cout.conditionId, [Cout.conditionDesc; uint8(0)], Cout.delayNominal);
    else
        coder.ceval('printf', ['C%d: %s delay %.0f ms [imaging active]' 10 0], ...
            Cout.conditionId, [Cout.conditionDesc; uint8(0)], Cout.delayNominal);
    end
end

end

== matlab function RefModel_Task/Condition Selection/Deserialize and Modify Selected Condition Once/Deserialize Element of Bus Array ==
  data: input input; bus output Bus: ConditionBus size=1; index input uint16 size=1; allowUpdate input uint8 size=1; receivedInvalid output uint8 size=1
function [bus, receivedInvalid] = deserializeBusArrayElement(input, index, allowUpdate)
%#codegen

    in = typecast(input, 'uint8');
    receivedInvalid = uint8(0);
    valid = uint8(0);

    % cached output for allowUpdate
    persistent pBus;
    
    % cache outputs so that we only update when allowUpdate is high
    if isempty(pBus)
        pBus = initializeBus_ConditionBus();        
    end
    
    % deserialize a new output if we're allowing updates
    if allowUpdate

        % length is first uint16
        N = typecast(in(1:2), 'uint16');
        if index <= N
            % followed by N uint32s indicating where each element starts
            idxOffset = uint32((index-1)*4 + 3); % first offset at byte 3, second at byte 7
            if idxOffset <= length(in) % too short to hold that many?
                % get the offset where the requested bus element starts
                offset = typecast(in(idxOffset : (idxOffset + 3)), 'uint32');
                if offset <= length(in) % offset invalid?

                    % and deserialize the bus from that offset
                    [bus, valid] = deserializeBus_ConditionBus(in, offset);
                    if valid
                        % cache as new output
                        pBus = bus;
                    end
                end
            end
        end

        if ~valid
            % don't update cache, restore old output
            receivedInvalid = uint8(1);
        end
    end

    bus = pBus;
end

== matlab function RefModel_Task/Condition Selection/Select Next Condition From Block ==
  data: chooseNewTrial input uint8 size=1; conditionRepeats input uint16 size=TaskInfo.maxConditions; randInt input uint32 size=1; preferNewCondition input; completedLastTrial input uint8 size=1; resetBlock input uint8 size=1; conditionSelected output uint16 size=1; nTrialsRemaining output uint16 size=1; blockComplete output uint8 size=1; TaskInfo parameter size=1
function [conditionSelected, nTrialsRemaining, blockComplete] = pseudorandomSelect(chooseNewTrial, conditionRepeats, ...
    randInt, preferNewCondition, completedLastTrial, resetBlock, TaskInfo)
%#codegen

% a MaxConditions array of repeats by condition, this is not variable size
% because of codegen bugs when variable sized persistents are used
persistent pRepeatsRemaining;

% scalar index into conditions array
persistent pConditionCurrent;

blockComplete = uint8(0);
nConditions = numel(conditionRepeats);

if isempty(pRepeatsRemaining) || resetBlock
    pRepeatsRemaining = zeros(TaskInfo.maxConditions, 1, 'uint16');
    pRepeatsRemaining(1:nConditions) = conditionRepeats;
    chooseNewTrial = uint8(1);
    completedLastTrial = uint8(0);
end

for i = 1:numel(conditionRepeats)
    if pRepeatsRemaining(i) > conditionRepeats(i)
        pRepeatsRemaining(i) = conditionRepeats(i);
    end
end

if isempty(pConditionCurrent)
    pConditionCurrent = uint16(1);
    chooseNewTrial = uint8(1);
    completedLastTrial = uint8(0);
end

% when chooseNewTrial is true, we'll pick a new trial
% this will have the same condition as the last one, unless
% prefer new condition is true, or the conditions have been updated or the
% block reset since the last trial was generated

% cache resets until new trial is generated
persistent pBlockHasBeenResetSinceLastTrial;
if isempty(pBlockHasBeenResetSinceLastTrial)
    pBlockHasBeenResetSinceLastTrial = false;
end
if resetBlock
    pBlockHasBeenResetSinceLastTrial = true;
end

% pick a new condition if block has been reset or we're asked for one
% explicitly
chooseNewCondition = pBlockHasBeenResetSinceLastTrial || preferNewCondition;

if completedLastTrial && chooseNewTrial
    % subtract one from the condition repeats number for the last
    % condition
    if pRepeatsRemaining(pConditionCurrent) > 0
        pRepeatsRemaining(pConditionCurrent) = pRepeatsRemaining(pConditionCurrent) - uint16(1);
        %coder.ceval('printf', ['now has reps = %d' 10 0], pRepeatsRemaining(pConditionCurrent));
    end
end
    
% compute number of trials remaining in block
nTrialsRemaining = uint16(0);
for i = 1:numel(pRepeatsRemaining);
    nTrialsRemaining = nTrialsRemaining + pRepeatsRemaining(i);
end

% pick a new condition pseudo-randomly looking at the pRepeatsRemaining
% lists
if chooseNewTrial && chooseNewCondition  
    pBlockHasBeenResetSinceLastTrial = false;
    
    % check whether we're starting a new block currently
    if nTrialsRemaining == uint16(0)
        % yes, reset the counts
        blockComplete = uint8(1);
        pRepeatsRemaining = zeros(TaskInfo.maxConditions, 1, 'like', conditionRepeats);
        pRepeatsRemaining(1:nConditions) = conditionRepeats;
        nTrialsRemaining = uint16(sum(pRepeatsRemaining));
    end
    
    % use the cumulative trial repetitions count (summing over conditions)
    % to choose a trial from the set of reps still to do
    selectorIdx = uint16(mod(randInt, uint32(nTrialsRemaining))) + 1;
    cumulativeReps = uint16(0);
    for iC = uint16(1):uint16(nConditions)
        cumulativeReps = cumulativeReps + uint16(pRepeatsRemaining(iC));
        if cumulativeReps >= selectorIdx
            pConditionCurrent = iC;
            break;
        end
    end
end

conditionSelected = pConditionCurrent;

== matlab function RefModel_Task/Condition Selection/Deserialize and Modify Selected Condition Once/Print Deserialization Alert ==
  data: active input size=1
function printAlert(active)

if active
    coder.ceval('printf', [char('Could not deserialize condition bus') 10 0]);
end

== matlab function RefModel_Task/Track Statistics ==
  data: trialEnd input uint8 size=1; trialData input Bus: TrialDataBus; taskStatistics output Bus: TaskStatisticsBus size=1; reset input uint8 size=1; trialsRemaining input size=1; blockCompleted input uint8 size=1
function taskStatistics = trackTaskStatistics(trialEnd, trialData, reset, trialsRemaining, blockCompleted)
%#codegen

persistent pSuccesses;
persistent pFailures;
persistent pBlocksCompleted;
if isempty(pSuccesses) || reset
    pSuccesses = uint16(0);
end
if isempty(pFailures) || reset
    pFailures = uint16(0);
end
if isempty(pBlocksCompleted) || reset
    pBlocksCompleted = uint16(0);
end

% recent moving average
persistent pHistory;
persistent pHistoryHead;
persistent pHistoryFilled;
nTrialsHistory = 100;
if isempty(pHistory) || isempty(pHistoryFilled) || reset
    pHistory = zeros(nTrialsHistory, 1, 'uint8');
    pHistoryFilled = uint16(0);
    pHistoryHead = uint16(1);
end

if trialEnd
    if trialData.success
        pSuccesses = pSuccesses + uint16(1);
    elseif trialData.substantiveFailure
        pFailures = pFailures + uint16(1);
    end
    
    % store this trial in moving average ring buffer
    if trialData.success || trialData.substantiveFailure
        pHistory(pHistoryHead) = trialData.success;
        pHistoryHead = pHistoryHead + uint16(1);
        if pHistoryHead > numel(pHistory)
            pHistoryHead = uint16(1);
        end
        pHistoryFilled = pHistoryFilled + uint16(1);
        if pHistoryHead > numel(pHistory)
            pHistoryHead = uint16(numel(pHistory));
        end
    end
end

if blockCompleted
    pBlocksCompleted = pBlocksCompleted + uint16(1);
end

taskStatistics = initializeBus_TaskStatisticsBus();
taskStatistics.successes = pSuccesses;
taskStatistics.failures = pFailures;
if pSuccesses + pFailures == 0
    taskStatistics.successRate = 0;
else
    taskStatistics.successRate = double(pSuccesses) / double(pSuccesses + pFailures);
end
if pHistoryFilled == 0
    taskStatistics.recentSuccessRate = 0;
else
    % we always fill from 1 on, pHistoryHead only loops around when
    % pHistoryFilled is saturated
    taskStatistics.recentSuccessRate = double(sum(pHistory(1:pHistoryFilled))) / double(pHistoryFilled);
end
taskStatistics.conditionBlockTrialsRemaining = trialsRemaining;
taskStatistics.conditionBlocksCompleted = pBlocksCompleted;

== matlab function RefModel_Task/Convert Condition Bus To Fixed ==
  data: bus input Bus: ConditionBus size=1; busFixed output Bus: ConditionFixedBus size=1
function busFixed = convertToConditionFixedBus(bus)
%#codegen

    busFixed = dropVariableLengthSignalsFromBus_ConditionBus(bus);

end
